simulink subsystem "EarthMagneticField_SS"  (R2023a)
settings: Solver=VariableStepAuto  StartTime=0.0  StopTime=10.0  RelTol=1e-3
undefined symbols (not defined in the file or in its folder): IAU, r0, WMM2020
libraries: aerolibtransform2 x1, aerolibgravity2 x1
settings Model: Creator=jself  LastModifiedBy=willb

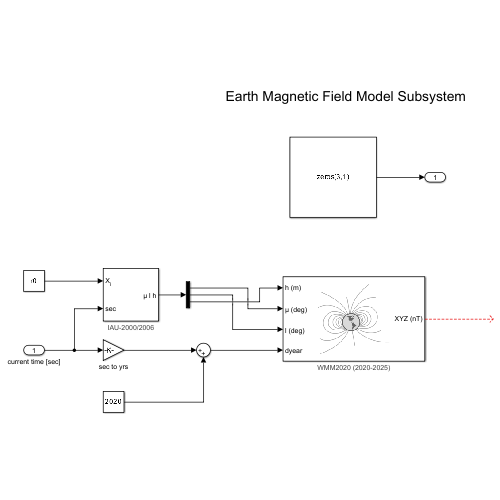
[thumbnail: Simulink's stored preview of the top-level diagram]
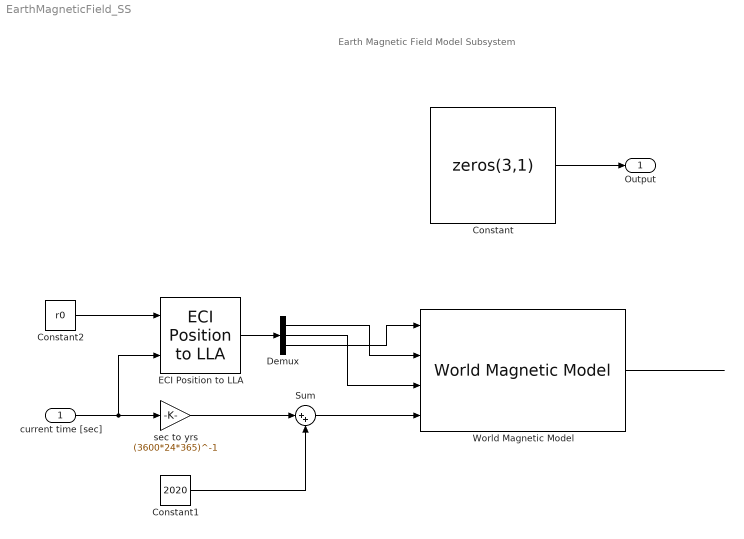
== system EarthMagneticField_SS ==
  note: Earth Magnetic Field Model Subsystem
  current time [sec] : Inport
  Constant : Constant  Value=zeros(3,1)
  Constant1 : Constant  Value=2020
  Constant2 : Constant  Value=r0
  Demux : Demux  Outputs=3
  ECI Position to LLA : aerolibtransform2/ECI Position to LLA  red=IAU-2000/2006  year=2020  month=January  day=1  hour=0  min=0  sec=0  deltaT=Sec  errorflag=Error  extraparamflag=off  eunits=Metric (MKS)  earthmodel=WGS84  flat=1/298.257223563  eqradius=6378137
      settings: AttributesFormatString=%<red>
  Sum : Sum  Inputs=|++
  World Magnetic Model : aerolibgravity2/World Magnetic Model  model=WMM2020 (2020-2025)  customFile='WMM2020.COF'  units=Metric (MKS)  time_in=on  month=January  day=1  year=2020  action=Error  h_out=off  dec_out=off  inc_out=off  ti_out=off
  sec to yrs : Gain  Gain=(3600*24*365)^-1
  Output : Outport
  wires:
  Constant/1 -> Output/1
  current time [sec]/1 -> ECI Position to LLA/2, sec to yrs/1
  sec to yrs/1 -> Sum/1
  Sum/1 -> World Magnetic Model/4
  Constant1/1 -> Sum/2
  Constant2/1 -> ECI Position to LLA/1
  ECI Position to LLA/1 -> Demux/1
  Demux/3 -> World Magnetic Model/1
  Demux/2 -> World Magnetic Model/3
  Demux/1 -> World Magnetic Model/2
  World Magnetic Model/1 -> ?
